simulink library "GOODVAL_MASTER"  (Simulink 8.6)
settings: Solver=ode45  StartTime=0.0  StopTime=10.0  RelTol=1e-3
libraries: cdsEpicsIn x174, GOODVAL_MASTER x17, cdsEpicsBinIn x6
(part 1 of 4)
settings Model: Creator=controls  LastModifiedBy=controls

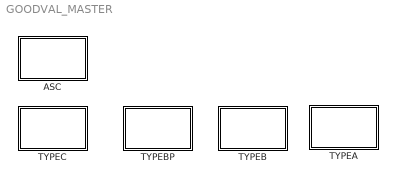
== system GOODVAL_MASTER ==
  ASC : Subsystem
  TYPEA : Subsystem
  TYPEB : Subsystem
  TYPEBP : Subsystem
  TYPEC : Subsystem

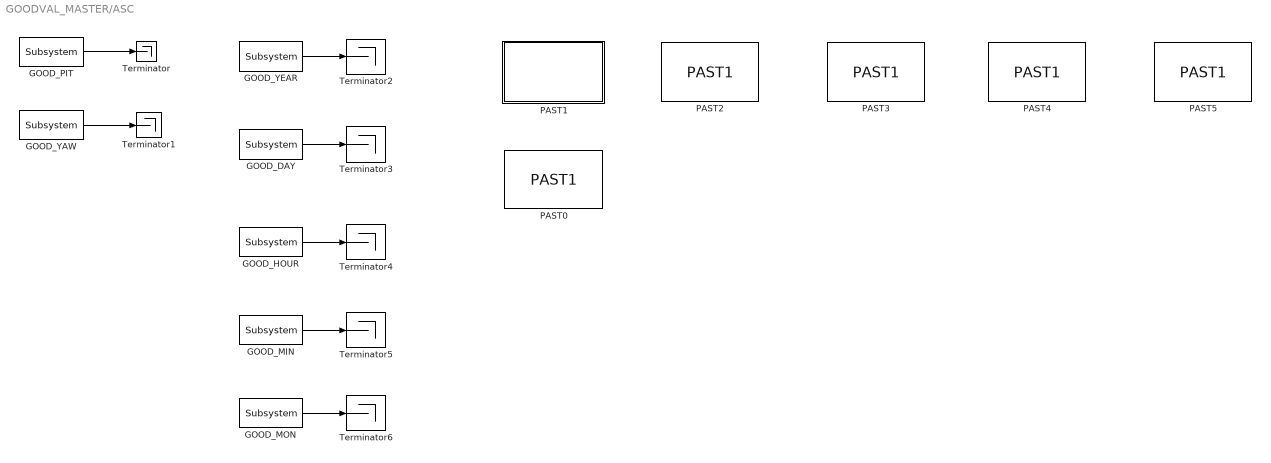
== system GOODVAL_MASTER/ASC ==
  GOOD_DAY : cdsEpicsIn/Subsystem  Tag=cdsEpicsIn  Description=|
      | Purpose:                                                                              
      | Create an EPICS input channel connection to the FE realtime controls.                 
      |                                                                                       
      | Operation:                                                                            
      | Outputs value from an EPICS ai record. Value is floating point with a precision of 3..
      |                                                                                       
      | Usage:                                                                                
      | Name the part with the desired EPICS channel name.
      settings: AttributesFormatString=%<Tag>
  GOOD_HOUR : cdsEpicsIn/Subsystem  Tag=cdsEpicsIn  Description=|
      | Purpose:                                                                              
      | Create an EPICS input channel connection to the FE realtime controls.                 
      |                                                                                       
      | Operation:                                                                            
      | Outputs value from an EPICS ai record. Value is floating point with a precision of 3..
      |                                                                                       
      | Usage:                                                                                
      | Name the part with the desired EPICS channel name.
      settings: AttributesFormatString=%<Tag>
  GOOD_MIN : cdsEpicsIn/Subsystem  Tag=cdsEpicsIn  Description=|
      | Purpose:                                                                              
      | Create an EPICS input channel connection to the FE realtime controls.                 
      |                                                                                       
      | Operation:                                                                            
      | Outputs value from an EPICS ai record. Value is floating point with a precision of 3..
      |                                                                                       
      | Usage:                                                                                
      | Name the part with the desired EPICS channel name.
      settings: AttributesFormatString=%<Tag>
  GOOD_MON : cdsEpicsIn/Subsystem  Tag=cdsEpicsIn  Description=|
      | Purpose:                                                                              
      | Create an EPICS input channel connection to the FE realtime controls.                 
      |                                                                                       
      | Operation:                                                                            
      | Outputs value from an EPICS ai record. Value is floating point with a precision of 3..
      |                                                                                       
      | Usage:                                                                                
      | Name the part with the desired EPICS channel name.
      settings: AttributesFormatString=%<Tag>
  GOOD_PIT : cdsEpicsIn/Subsystem  Tag=cdsEpicsIn  Description=|
      | Purpose:                                                                              
      | Create an EPICS input channel connection to the FE realtime controls.                 
      |                                                                                       
      | Operation:                                                                            
      | Outputs value from an EPICS ai record. Value is floating point with a precision of 3..
      |                                                                                       
      | Usage:                                                                                
      | Name the part with the desired EPICS channel name.
      settings: AttributesFormatString=%<Tag>
  GOOD_YAW : cdsEpicsIn/Subsystem  Tag=cdsEpicsIn  Description=|
      | Purpose:                                                                              
      | Create an EPICS input channel connection to the FE realtime controls.                 
      |                                                                                       
      | Operation:                                                                            
      | Outputs value from an EPICS ai record. Value is floating point with a precision of 3..
      |                                                                                       
      | Usage:                                                                                
      | Name the part with the desired EPICS channel name.
      settings: AttributesFormatString=%<Tag>
  GOOD_YEAR : cdsEpicsIn/Subsystem  Tag=cdsEpicsIn  Description=|
      | Purpose:                                                                              
      | Create an EPICS input channel connection to the FE realtime controls.                 
      |                                                                                       
      | Operation:                                                                            
      | Outputs value from an EPICS ai record. Value is floating point with a precision of 3..
      |                                                                                       
      | Usage:                                                                                
      | Name the part with the desired EPICS channel name.
      settings: AttributesFormatString=%<Tag>
  PAST{0,2..5} (5 alike) : GOODVAL_MASTER/ASC/PAST1
  PAST1 : Subsystem
  Terminator{,1..6} (7 alike) : Terminator
  wires:
  GOOD_PIT/1 -> Terminator/1
  GOOD_YAW/1 -> Terminator1/1
  GOOD_YEAR/1 -> Terminator2/1
  GOOD_DAY/1 -> Terminator3/1
  GOOD_HOUR/1 -> Terminator4/1
  GOOD_MIN/1 -> Terminator5/1
  GOOD_MON/1 -> Terminator6/1

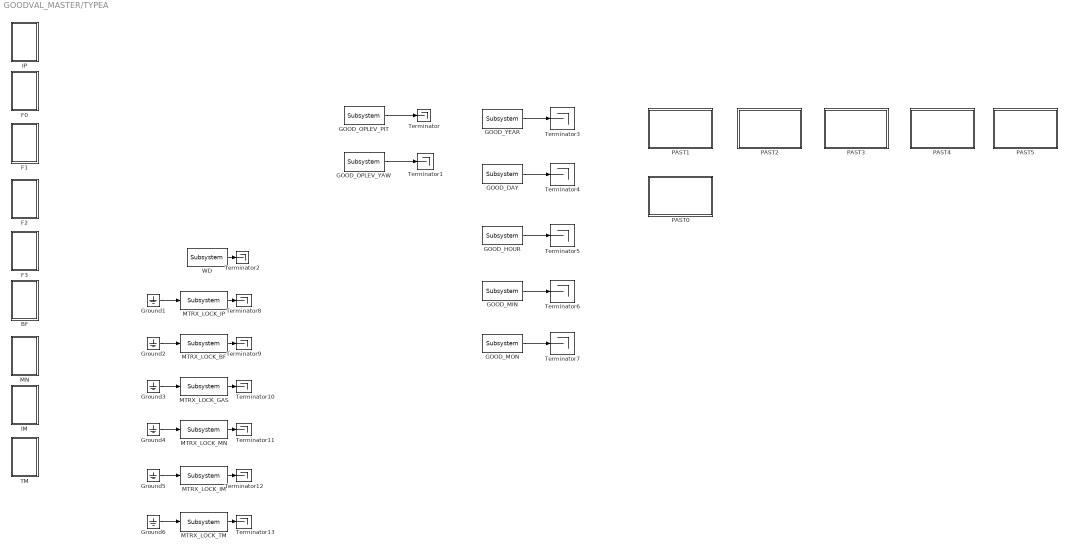
== system GOODVAL_MASTER/TYPEA ==
  BF : Subsystem
  F0 : Subsystem
  F1 : Subsystem
  F2 : Subsystem
  F3 : Subsystem
  GOOD_DAY : cdsEpicsIn/Subsystem  Tag=cdsEpicsIn  Description=|
      | Purpose:                                                                              
      | Create an EPICS input channel connection to the FE realtime controls.                 
      |                                                                                       
      | Operation:                                                                            
      | Outputs value from an EPICS ai record. Value is floating point with a precision of 3..
      |                                                                                       
      | Usage:                                                                                
      | Name the part with the desired EPICS channel name.
      settings: AttributesFormatString=%<Tag>
  GOOD_HOUR : cdsEpicsIn/Subsystem  Tag=cdsEpicsIn  Description=|
      | Purpose:                                                                              
      | Create an EPICS input channel connection to the FE realtime controls.                 
      |                                                                                       
      | Operation:                                                                            
      | Outputs value from an EPICS ai record. Value is floating point with a precision of 3..
      |                                                                                       
      | Usage:                                                                                
      | Name the part with the desired EPICS channel name.
      settings: AttributesFormatString=%<Tag>
  GOOD_MIN : cdsEpicsIn/Subsystem  Tag=cdsEpicsIn  Description=|
      | Purpose:                                                                              
      | Create an EPICS input channel connection to the FE realtime controls.                 
      |                                                                                       
      | Operation:                                                                            
      | Outputs value from an EPICS ai record. Value is floating point with a precision of 3..
      |                                                                                       
      | Usage:                                                                                
      | Name the part with the desired EPICS channel name.
      settings: AttributesFormatString=%<Tag>
  GOOD_MON : cdsEpicsIn/Subsystem  Tag=cdsEpicsIn  Description=|
      | Purpose:                                                                              
      | Create an EPICS input channel connection to the FE realtime controls.                 
      |                                                                                       
      | Operation:                                                                            
      | Outputs value from an EPICS ai record. Value is floating point with a precision of 3..
      |                                                                                       
      | Usage:                                                                                
      | Name the part with the desired EPICS channel name.
      settings: AttributesFormatString=%<Tag>
  GOOD_OPLEV_PIT : cdsEpicsIn/Subsystem  Tag=cdsEpicsIn  Description=|
      | Purpose:                                                                              
      | Create an EPICS input channel connection to the FE realtime controls.                 
      |                                                                                       
      | Operation:                                                                            
      | Outputs value from an EPICS ai record. Value is floating point with a precision of 3..
      |                                                                                       
      | Usage:                                                                                
      | Name the part with the desired EPICS channel name.
      settings: AttributesFormatString=%<Tag>
  GOOD_OPLEV_YAW : cdsEpicsIn/Subsystem  Tag=cdsEpicsIn  Description=|
      | Purpose:                                                                              
      | Create an EPICS input channel connection to the FE realtime controls.                 
      |                                                                                       
      | Operation:                                                                            
      | Outputs value from an EPICS ai record. Value is floating point with a precision of 3..
      |                                                                                       
      | Usage:                                                                                
      | Name the part with the desired EPICS channel name.
      settings: AttributesFormatString=%<Tag>
  GOOD_YEAR : cdsEpicsIn/Subsystem  Tag=cdsEpicsIn  Description=|
      | Purpose:                                                                              
      | Create an EPICS input channel connection to the FE realtime controls.                 
      |                                                                                       
      | Operation:                                                                            
      | Outputs value from an EPICS ai record. Value is floating point with a precision of 3..
      |                                                                                       
      | Usage:                                                                                
      | Name the part with the desired EPICS channel name.
      settings: AttributesFormatString=%<Tag>
  Ground{1..6} (6 alike) : Ground
  IM : Subsystem
  IP : Subsystem
  MN : Subsystem
  MTRX_LOCK_BF : cdsEpicsBinIn/Subsystem  Tag=cdsEpicsBinIn  Description=|
      | Purpose:                                                                            
      | Create an EPICS binary (0 or 1) input channel to the FE realtime controls.          
      |                                                                                     
      | Operation:                                                                          
      | Outputs value from an EPICS ai record. Value is binary input (bi Epics record type).
      |                                                                                     
      | Usage:                                                                              
      | Name the part with the desired EPICS channel name.
      settings: AttributesFormatString=%<Tag>
  MTRX_LOCK_GAS : cdsEpicsBinIn/Subsystem  Tag=cdsEpicsBinIn  Description=|
      | Purpose:                                                                            
      | Create an EPICS binary (0 or 1) input channel to the FE realtime controls.          
      |                                                                                     
      | Operation:                                                                          
      | Outputs value from an EPICS ai record. Value is binary input (bi Epics record type).
      |                                                                                     
      | Usage:                                                                              
      | Name the part with the desired EPICS channel name.
      settings: AttributesFormatString=%<Tag>
  MTRX_LOCK_IM : cdsEpicsBinIn/Subsystem  Tag=cdsEpicsBinIn  Description=|
      | Purpose:                                                                            
      | Create an EPICS binary (0 or 1) input channel to the FE realtime controls.          
      |                                                                                     
      | Operation:                                                                          
      | Outputs value from an EPICS ai record. Value is binary input (bi Epics record type).
      |                                                                                     
      | Usage:                                                                              
      | Name the part with the desired EPICS channel name.
      settings: AttributesFormatString=%<Tag>
  MTRX_LOCK_IP : cdsEpicsBinIn/Subsystem  Tag=cdsEpicsBinIn  Description=|
      | Purpose:                                                                            
      | Create an EPICS binary (0 or 1) input channel to the FE realtime controls.          
      |                                                                                     
      | Operation:                                                                          
      | Outputs value from an EPICS ai record. Value is binary input (bi Epics record type).
      |                                                                                     
      | Usage:                                                                              
      | Name the part with the desired EPICS channel name.
      settings: AttributesFormatString=%<Tag>
  MTRX_LOCK_MN : cdsEpicsBinIn/Subsystem  Tag=cdsEpicsBinIn  Description=|
      | Purpose:                                                                            
      | Create an EPICS binary (0 or 1) input channel to the FE realtime controls.          
      |                                                                                     
      | Operation:                                                                          
      | Outputs value from an EPICS ai record. Value is binary input (bi Epics record type).
      |                                                                                     
      | Usage:                                                                              
      | Name the part with the desired EPICS channel name.
      settings: AttributesFormatString=%<Tag>
  MTRX_LOCK_TM : cdsEpicsBinIn/Subsystem  Tag=cdsEpicsBinIn  Description=|
      | Purpose:                                                                            
      | Create an EPICS binary (0 or 1) input channel to the FE realtime controls.          
      |                                                                                     
      | Operation:                                                                          
      | Outputs value from an EPICS ai record. Value is binary input (bi Epics record type).
      |                                                                                     
      | Usage:                                                                              
      | Name the part with the desired EPICS channel name.
      settings: AttributesFormatString=%<Tag>
  PAST0 : Subsystem
  PAST1 : Subsystem
  PAST2 : Subsystem
  PAST3 : Subsystem
  PAST4 : Subsystem
  PAST5 : Subsystem
  TM : Subsystem
  Terminator{,1..13} (14 alike) : Terminator
  WD : cdsEpicsIn/Subsystem  Tag=cdsEpicsIn  Description=|
      | Purpose:                                                                              
      | Create an EPICS input channel connection to the FE realtime controls.                 
      |                                                                                       
      | Operation:                                                                            
      | Outputs value from an EPICS ai record. Value is floating point with a precision of 3..
      |                                                                                       
      | Usage:                                                                                
      | Name the part with the desired EPICS channel name.
      settings: AttributesFormatString=%<Tag>
  wires:
  MTRX_LOCK_TM/1 -> Terminator13/1
  Ground6/1 -> MTRX_LOCK_TM/1
  MTRX_LOCK_IM/1 -> Terminator12/1
  Ground5/1 -> MTRX_LOCK_IM/1
  MTRX_LOCK_MN/1 -> Terminator11/1
  Ground4/1 -> MTRX_LOCK_MN/1
  MTRX_LOCK_GAS/1 -> Terminator10/1
  Ground3/1 -> MTRX_LOCK_GAS/1
  Ground2/1 -> MTRX_LOCK_BF/1
  MTRX_LOCK_BF/1 -> Terminator9/1
  Ground1/1 -> MTRX_LOCK_IP/1
  MTRX_LOCK_IP/1 -> Terminator8/1
  GOOD_OPLEV_PIT/1 -> Terminator/1
  GOOD_OPLEV_YAW/1 -> Terminator1/1
  GOOD_YEAR/1 -> Terminator3/1
  GOOD_DAY/1 -> Terminator4/1
  GOOD_HOUR/1 -> Terminator5/1
  GOOD_MIN/1 -> Terminator6/1
  GOOD_MON/1 -> Terminator7/1
  WD/1 -> Terminator2/1

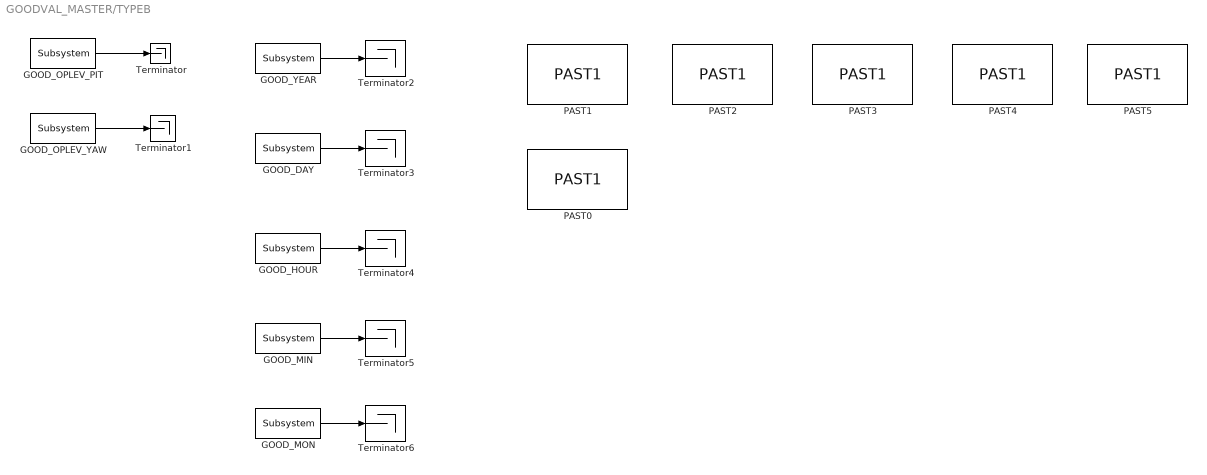
== system GOODVAL_MASTER/TYPEB ==
  GOOD_DAY : cdsEpicsIn/Subsystem  Tag=cdsEpicsIn  Description=|
      | Purpose:                                                                              
      | Create an EPICS input channel connection to the FE realtime controls.                 
      |                                                                                       
      | Operation:                                                                            
      | Outputs value from an EPICS ai record. Value is floating point with a precision of 3..
      |                                                                                       
      | Usage:                                                                                
      | Name the part with the desired EPICS channel name.
      settings: AttributesFormatString=%<Tag>
  GOOD_HOUR : cdsEpicsIn/Subsystem  Tag=cdsEpicsIn  Description=|
      | Purpose:                                                                              
      | Create an EPICS input channel connection to the FE realtime controls.                 
      |                                                                                       
      | Operation:                                                                            
      | Outputs value from an EPICS ai record. Value is floating point with a precision of 3..
      |                                                                                       
      | Usage:                                                                                
      | Name the part with the desired EPICS channel name.
      settings: AttributesFormatString=%<Tag>
  GOOD_MIN : cdsEpicsIn/Subsystem  Tag=cdsEpicsIn  Description=|
      | Purpose:                                                                              
      | Create an EPICS input channel connection to the FE realtime controls.                 
      |                                                                                       
      | Operation:                                                                            
      | Outputs value from an EPICS ai record. Value is floating point with a precision of 3..
      |                                                                                       
      | Usage:                                                                                
      | Name the part with the desired EPICS channel name.
      settings: AttributesFormatString=%<Tag>
  GOOD_MON : cdsEpicsIn/Subsystem  Tag=cdsEpicsIn  Description=|
      | Purpose:                                                                              
      | Create an EPICS input channel connection to the FE realtime controls.                 
      |                                                                                       
      | Operation:                                                                            
      | Outputs value from an EPICS ai record. Value is floating point with a precision of 3..
      |                                                                                       
      | Usage:                                                                                
      | Name the part with the desired EPICS channel name.
      settings: AttributesFormatString=%<Tag>
  GOOD_OPLEV_PIT : cdsEpicsIn/Subsystem  Tag=cdsEpicsIn  Description=|
      | Purpose:                                                                              
      | Create an EPICS input channel connection to the FE realtime controls.                 
      |                                                                                       
      | Operation:                                                                            
      | Outputs value from an EPICS ai record. Value is floating point with a precision of 3..
      |                                                                                       
      | Usage:                                                                                
      | Name the part with the desired EPICS channel name.
      settings: AttributesFormatString=%<Tag>
  GOOD_OPLEV_YAW : cdsEpicsIn/Subsystem  Tag=cdsEpicsIn  Description=|
      | Purpose:                                                                              
      | Create an EPICS input channel connection to the FE realtime controls.                 
      |                                                                                       
      | Operation:                                                                            
      | Outputs value from an EPICS ai record. Value is floating point with a precision of 3..
      |                                                                                       
      | Usage:                                                                                
      | Name the part with the desired EPICS channel name.
      settings: AttributesFormatString=%<Tag>
  GOOD_YEAR : cdsEpicsIn/Subsystem  Tag=cdsEpicsIn  Description=|
      | Purpose:                                                                              
      | Create an EPICS input channel connection to the FE realtime controls.                 
      |                                                                                       
      | Operation:                                                                            
      | Outputs value from an EPICS ai record. Value is floating point with a precision of 3..
      |                                                                                       
      | Usage:                                                                                
      | Name the part with the desired EPICS channel name.
      settings: AttributesFormatString=%<Tag>
  PAST{0..5} (6 alike) : GOODVAL_MASTER/TYPEC/PAST1
  Terminator{,1..6} (7 alike) : Terminator
  wires:
  GOOD_OPLEV_PIT/1 -> Terminator/1
  GOOD_OPLEV_YAW/1 -> Terminator1/1
  GOOD_YEAR/1 -> Terminator2/1
  GOOD_DAY/1 -> Terminator3/1
  GOOD_HOUR/1 -> Terminator4/1
  GOOD_MIN/1 -> Terminator5/1
  GOOD_MON/1 -> Terminator6/1

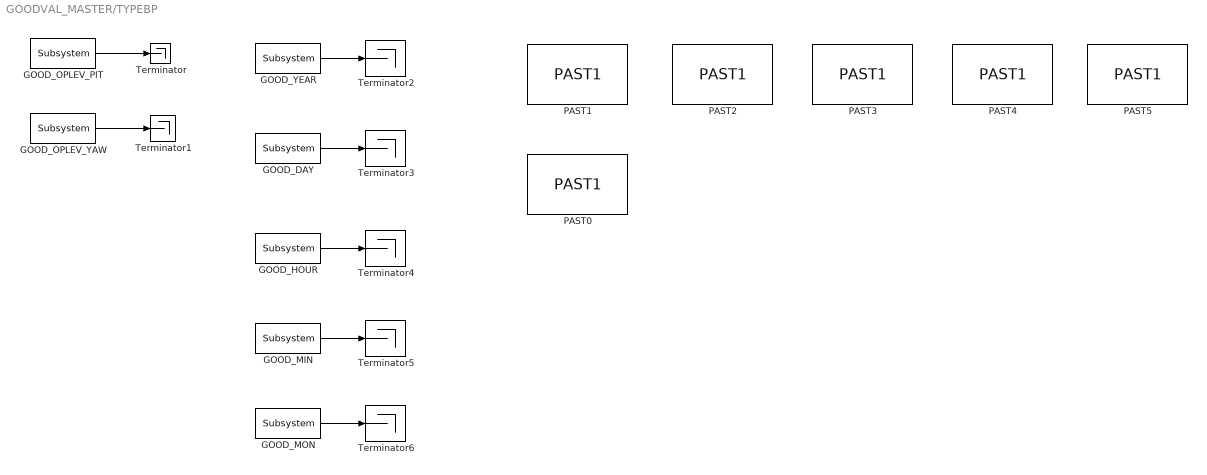
== system GOODVAL_MASTER/TYPEBP ==
  GOOD_DAY : cdsEpicsIn/Subsystem  Tag=cdsEpicsIn  Description=|
      | Purpose:                                                                              
      | Create an EPICS input channel connection to the FE realtime controls.                 
      |                                                                                       
      | Operation:                                                                            
      | Outputs value from an EPICS ai record. Value is floating point with a precision of 3..
      |                                                                                       
      | Usage:                                                                                
      | Name the part with the desired EPICS channel name.
      settings: AttributesFormatString=%<Tag>
  GOOD_HOUR : cdsEpicsIn/Subsystem  Tag=cdsEpicsIn  Description=|
      | Purpose:                                                                              
      | Create an EPICS input channel connection to the FE realtime controls.                 
      |                                                                                       
      | Operation:                                                                            
      | Outputs value from an EPICS ai record. Value is floating point with a precision of 3..
      |                                                                                       
      | Usage:                                                                                
      | Name the part with the desired EPICS channel name.
      settings: AttributesFormatString=%<Tag>
  GOOD_MIN : cdsEpicsIn/Subsystem  Tag=cdsEpicsIn  Description=|
      | Purpose:                                                                              
      | Create an EPICS input channel connection to the FE realtime controls.                 
      |                                                                                       
      | Operation:                                                                            
      | Outputs value from an EPICS ai record. Value is floating point with a precision of 3..
      |                                                                                       
      | Usage:                                                                                
      | Name the part with the desired EPICS channel name.
      settings: AttributesFormatString=%<Tag>
  GOOD_MON : cdsEpicsIn/Subsystem  Tag=cdsEpicsIn  Description=|
      | Purpose:                                                                              
      | Create an EPICS input channel connection to the FE realtime controls.                 
      |                                                                                       
      | Operation:                                                                            
      | Outputs value from an EPICS ai record. Value is floating point with a precision of 3..
      |                                                                                       
      | Usage:                                                                                
      | Name the part with the desired EPICS channel name.
      settings: AttributesFormatString=%<Tag>
  GOOD_OPLEV_PIT : cdsEpicsIn/Subsystem  Tag=cdsEpicsIn  Description=|
      | Purpose:                                                                              
      | Create an EPICS input channel connection to the FE realtime controls.                 
      |                                                                                       
      | Operation:                                                                            
      | Outputs value from an EPICS ai record. Value is floating point with a precision of 3..
      |                                                                                       
      | Usage:                                                                                
      | Name the part with the desired EPICS channel name.
      settings: AttributesFormatString=%<Tag>
  GOOD_OPLEV_YAW : cdsEpicsIn/Subsystem  Tag=cdsEpicsIn  Description=|
      | Purpose:                                                                              
      | Create an EPICS input channel connection to the FE realtime controls.                 
      |                                                                                       
      | Operation:                                                                            
      | Outputs value from an EPICS ai record. Value is floating point with a precision of 3..
      |                                                                                       
      | Usage:                                                                                
      | Name the part with the desired EPICS channel name.
      settings: AttributesFormatString=%<Tag>
  GOOD_YEAR : cdsEpicsIn/Subsystem  Tag=cdsEpicsIn  Description=|
      | Purpose:                                                                              
      | Create an EPICS input channel connection to the FE realtime controls.                 
      |                                                                                       
      | Operation:                                                                            
      | Outputs value from an EPICS ai record. Value is floating point with a precision of 3..
      |                                                                                       
      | Usage:                                                                                
      | Name the part with the desired EPICS channel name.
      settings: AttributesFormatString=%<Tag>
  PAST{0..5} (6 alike) : GOODVAL_MASTER/TYPEC/PAST1
  Terminator{,1..6} (7 alike) : Terminator
  wires:
  GOOD_OPLEV_PIT/1 -> Terminator/1
  GOOD_OPLEV_YAW/1 -> Terminator1/1
  GOOD_YEAR/1 -> Terminator2/1
  GOOD_DAY/1 -> Terminator3/1
  GOOD_HOUR/1 -> Terminator4/1
  GOOD_MIN/1 -> Terminator5/1
  GOOD_MON/1 -> Terminator6/1

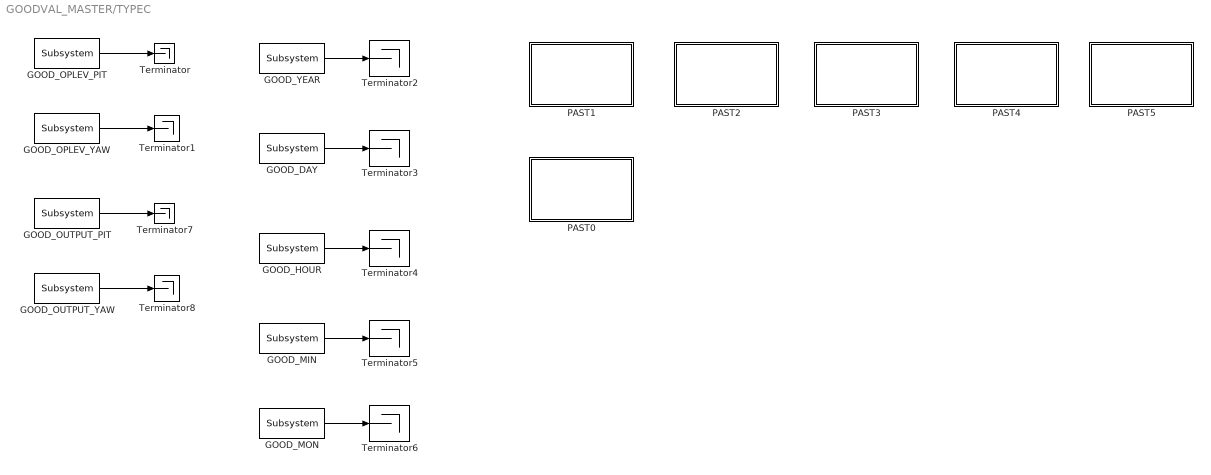
== system GOODVAL_MASTER/TYPEC ==
  GOOD_DAY : cdsEpicsIn/Subsystem  Tag=cdsEpicsIn  Description=|
      | Purpose:                                                                              
      | Create an EPICS input channel connection to the FE realtime controls.                 
      |                                                                                       
      | Operation:                                                                            
      | Outputs value from an EPICS ai record. Value is floating point with a precision of 3..
      |                                                                                       
      | Usage:                                                                                
      | Name the part with the desired EPICS channel name.
      settings: AttributesFormatString=%<Tag>
  GOOD_HOUR : cdsEpicsIn/Subsystem  Tag=cdsEpicsIn  Description=|
      | Purpose:                                                                              
      | Create an EPICS input channel connection to the FE realtime controls.                 
      |                                                                                       
      | Operation:                                                                            
      | Outputs value from an EPICS ai record. Value is floating point with a precision of 3..
      |                                                                                       
      | Usage:                                                                                
      | Name the part with the desired EPICS channel name.
      settings: AttributesFormatString=%<Tag>
  GOOD_MIN : cdsEpicsIn/Subsystem  Tag=cdsEpicsIn  Description=|
      | Purpose:                                                                              
      | Create an EPICS input channel connection to the FE realtime controls.                 
      |                                                                                       
      | Operation:                                                                            
      | Outputs value from an EPICS ai record. Value is floating point with a precision of 3..
      |                                                                                       
      | Usage:                                                                                
      | Name the part with the desired EPICS channel name.
      settings: AttributesFormatString=%<Tag>
  GOOD_MON : cdsEpicsIn/Subsystem  Tag=cdsEpicsIn  Description=|
      | Purpose:                                                                              
      | Create an EPICS input channel connection to the FE realtime controls.                 
      |                                                                                       
      | Operation:                                                                            
      | Outputs value from an EPICS ai record. Value is floating point with a precision of 3..
      |                                                                                       
      | Usage:                                                                                
      | Name the part with the desired EPICS channel name.
      settings: AttributesFormatString=%<Tag>
  GOOD_OPLEV_PIT : cdsEpicsIn/Subsystem  Tag=cdsEpicsIn  Description=|
      | Purpose:                                                                              
      | Create an EPICS input channel connection to the FE realtime controls.                 
      |                                                                                       
      | Operation:                                                                            
      | Outputs value from an EPICS ai record. Value is floating point with a precision of 3..
      |                                                                                       
      | Usage:                                                                                
      | Name the part with the desired EPICS channel name.
      settings: AttributesFormatString=%<Tag>
  GOOD_OPLEV_YAW : cdsEpicsIn/Subsystem  Tag=cdsEpicsIn  Description=|
      | Purpose:                                                                              
      | Create an EPICS input channel connection to the FE realtime controls.                 
      |                                                                                       
      | Operation:                                                                            
      | Outputs value from an EPICS ai record. Value is floating point with a precision of 3..
      |                                                                                       
      | Usage:                                                                                
      | Name the part with the desired EPICS channel name.
      settings: AttributesFormatString=%<Tag>
  GOOD_OUTPUT_PIT : cdsEpicsIn/Subsystem  Tag=cdsEpicsIn  Description=|
      | Purpose:                                                                              
      | Create an EPICS input channel connection to the FE realtime controls.                 
      |                                                                                       
      | Operation:                                                                            
      | Outputs value from an EPICS ai record. Value is floating point with a precision of 3..
      |                                                                                       
      | Usage:                                                                                
      | Name the part with the desired EPICS channel name.
      settings: AttributesFormatString=%<Tag>
  GOOD_OUTPUT_YAW : cdsEpicsIn/Subsystem  Tag=cdsEpicsIn  Description=|
      | Purpose:                                                                              
      | Create an EPICS input channel connection to the FE realtime controls.                 
      |                                                                                       
      | Operation:                                                                            
      | Outputs value from an EPICS ai record. Value is floating point with a precision of 3..
      |                                                                                       
      | Usage:                                                                                
      | Name the part with the desired EPICS channel name.
      settings: AttributesFormatString=%<Tag>
  GOOD_YEAR : cdsEpicsIn/Subsystem  Tag=cdsEpicsIn  Description=|
      | Purpose:                                                                              
      | Create an EPICS input channel connection to the FE realtime controls.                 
      |                                                                                       
      | Operation:                                                                            
      | Outputs value from an EPICS ai record. Value is floating point with a precision of 3..
      |                                                                                       
      | Usage:                                                                                
      | Name the part with the desired EPICS channel name.
      settings: AttributesFormatString=%<Tag>
  PAST0 : Subsystem
  PAST1 : Subsystem
  PAST2 : Subsystem
  PAST3 : Subsystem
  PAST4 : Subsystem
  PAST5 : Subsystem
  Terminator{,1..8} (9 alike) : Terminator
  wires:
  GOOD_OUTPUT_PIT/1 -> Terminator7/1
  GOOD_OUTPUT_YAW/1 -> Terminator8/1
  GOOD_OPLEV_PIT/1 -> Terminator/1
  GOOD_OPLEV_YAW/1 -> Terminator1/1
  GOOD_YEAR/1 -> Terminator2/1
  GOOD_DAY/1 -> Terminator3/1
  GOOD_HOUR/1 -> Terminator4/1
  GOOD_MIN/1 -> Terminator5/1
  GOOD_MON/1 -> Terminator6/1

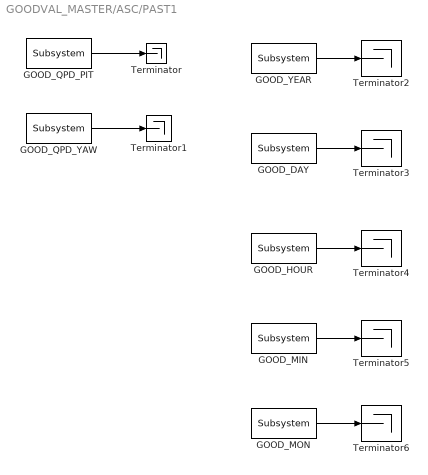
== system GOODVAL_MASTER/ASC/PAST1 ==
  GOOD_DAY : cdsEpicsIn/Subsystem  Tag=cdsEpicsIn  Description=|
      | Purpose:                                                                              
      | Create an EPICS input channel connection to the FE realtime controls.                 
      |                                                                                       
      | Operation:                                                                            
      | Outputs value from an EPICS ai record. Value is floating point with a precision of 3..
      |                                                                                       
      | Usage:                                                                                
      | Name the part with the desired EPICS channel name.
      settings: AttributesFormatString=%<Tag>
  GOOD_HOUR : cdsEpicsIn/Subsystem  Tag=cdsEpicsIn  Description=|
      | Purpose:                                                                              
      | Create an EPICS input channel connection to the FE realtime controls.                 
      |                                                                                       
      | Operation:                                                                            
      | Outputs value from an EPICS ai record. Value is floating point with a precision of 3..
      |                                                                                       
      | Usage:                                                                                
      | Name the part with the desired EPICS channel name.
      settings: AttributesFormatString=%<Tag>
  GOOD_MIN : cdsEpicsIn/Subsystem  Tag=cdsEpicsIn  Description=|
      | Purpose:                                                                              
      | Create an EPICS input channel connection to the FE realtime controls.                 
      |                                                                                       
      | Operation:                                                                            
      | Outputs value from an EPICS ai record. Value is floating point with a precision of 3..
      |                                                                                       
      | Usage:                                                                                
      | Name the part with the desired EPICS channel name.
      settings: AttributesFormatString=%<Tag>
  GOOD_MON : cdsEpicsIn/Subsystem  Tag=cdsEpicsIn  Description=|
      | Purpose:                                                                              
      | Create an EPICS input channel connection to the FE realtime controls.                 
      |                                                                                       
      | Operation:                                                                            
      | Outputs value from an EPICS ai record. Value is floating point with a precision of 3..
      |                                                                                       
      | Usage:                                                                                
      | Name the part with the desired EPICS channel name.
      settings: AttributesFormatString=%<Tag>
  GOOD_QPD_PIT : cdsEpicsIn/Subsystem  Tag=cdsEpicsIn  Description=|
      | Purpose:                                                                              
      | Create an EPICS input channel connection to the FE realtime controls.                 
      |                                                                                       
      | Operation:                                                                            
      | Outputs value from an EPICS ai record. Value is floating point with a precision of 3..
      |                                                                                       
      | Usage:                                                                                
      | Name the part with the desired EPICS channel name.
      settings: AttributesFormatString=%<Tag>
  GOOD_QPD_YAW : cdsEpicsIn/Subsystem  Tag=cdsEpicsIn  Description=|
      | Purpose:                                                                              
      | Create an EPICS input channel connection to the FE realtime controls.                 
      |                                                                                       
      | Operation:                                                                            
      | Outputs value from an EPICS ai record. Value is floating point with a precision of 3..
      |                                                                                       
      | Usage:                                                                                
      | Name the part with the desired EPICS channel name.
      settings: AttributesFormatString=%<Tag>
  GOOD_YEAR : cdsEpicsIn/Subsystem  Tag=cdsEpicsIn  Description=|
      | Purpose:                                                                              
      | Create an EPICS input channel connection to the FE realtime controls.                 
      |                                                                                       
      | Operation:                                                                            
      | Outputs value from an EPICS ai record. Value is floating point with a precision of 3..
      |                                                                                       
      | Usage:                                                                                
      | Name the part with the desired EPICS channel name.
      settings: AttributesFormatString=%<Tag>
  Terminator{,1..6} (7 alike) : Terminator
  wires:
  GOOD_MIN/1 -> Terminator5/1
  GOOD_DAY/1 -> Terminator3/1
  GOOD_HOUR/1 -> Terminator4/1
  GOOD_MON/1 -> Terminator6/1
  GOOD_YEAR/1 -> Terminator2/1
  GOOD_QPD_PIT/1 -> Terminator/1
  GOOD_QPD_YAW/1 -> Terminator1/1

== system GOODVAL_MASTER/TYPEA/BF ==
  INMON : cdsEpicsIn/Subsystem  Tag=cdsEpicsIn  Description=|
      | Purpose:                                                                              
      | Create an EPICS input channel connection to the FE realtime controls.                 
      |                                                                                       
      | Operation:                                                                            
      | Outputs value from an EPICS ai record. Value is floating point with a precision of 3..
      |                                                                                       
      | Usage:                                                                                
      | Name the part with the desired EPICS channel name.
      settings: AttributesFormatString=%<Tag>
  OUTMON : cdsEpicsIn/Subsystem  Tag=cdsEpicsIn  Description=|
      | Purpose:                                                                              
      | Create an EPICS input channel connection to the FE realtime controls.                 
      |                                                                                       
      | Operation:                                                                            
      | Outputs value from an EPICS ai record. Value is floating point with a precision of 3..
      |                                                                                       
      | Usage:                                                                                
      | Name the part with the desired EPICS channel name.
      settings: AttributesFormatString=%<Tag>
  Terminator1 : Terminator
  Terminator2 : Terminator
  wires:
  INMON/1 -> Terminator1/1
  OUTMON/1 -> Terminator2/1

== system GOODVAL_MASTER/TYPEA/F0 ==
  INMON : cdsEpicsIn/Subsystem  Tag=cdsEpicsIn  Description=|
      | Purpose:                                                                              
      | Create an EPICS input channel connection to the FE realtime controls.                 
      |                                                                                       
      | Operation:                                                                            
      | Outputs value from an EPICS ai record. Value is floating point with a precision of 3..
      |                                                                                       
      | Usage:                                                                                
      | Name the part with the desired EPICS channel name.
      settings: AttributesFormatString=%<Tag>
  OUTMON : cdsEpicsIn/Subsystem  Tag=cdsEpicsIn  Description=|
      | Purpose:                                                                              
      | Create an EPICS input channel connection to the FE realtime controls.                 
      |                                                                                       
      | Operation:                                                                            
      | Outputs value from an EPICS ai record. Value is floating point with a precision of 3..
      |                                                                                       
      | Usage:                                                                                
      | Name the part with the desired EPICS channel name.
      settings: AttributesFormatString=%<Tag>
  Terminator1 : Terminator
  Terminator2 : Terminator
  wires:
  INMON/1 -> Terminator1/1
  OUTMON/1 -> Terminator2/1
